simulink model "Fake_Algorithm_Control"  (Simulink 7.5)
settings: Solver=ode45  StartTime=0.0  StopTime=10.0  RelTol=1e-3
undefined symbols (not defined in the file): ctrller
settings Model: Creator=sriddle  LastModifiedBy=sriddle

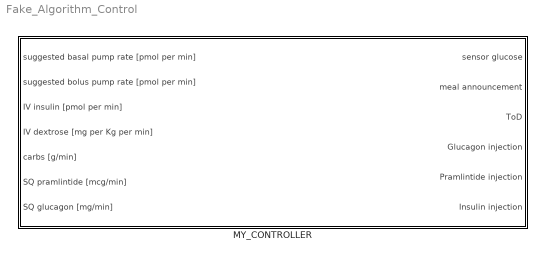
== system Fake_Algorithm_Control ==
  MY_CONTROLLER : Subsystem

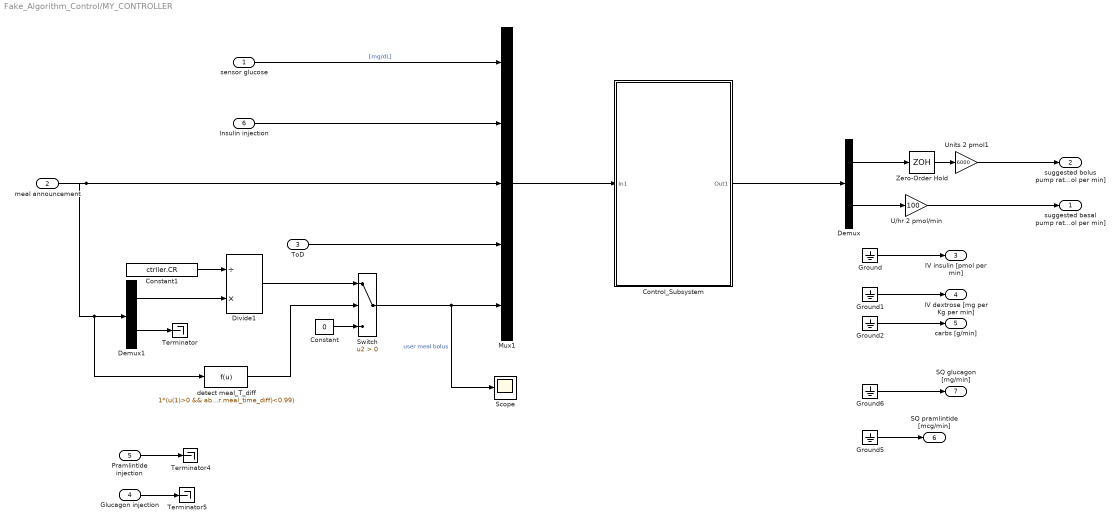
== system Fake_Algorithm_Control/MY_CONTROLLER ==
  sensor glucose : Inport  OutDataType=sfix(16)  OutScaling=2^0
  meal announcement : Inport  Port=2  OutDataType=sfix(16)  OutScaling=2^0
  ToD : Inport  Port=3  OutDataType=sfix(16)  OutScaling=2^0
  Glucagon injection : Inport  Port=4
  Pramlintide injection : Inport  Port=5
  Insulin injection : Inport  Port=6  OutDataType=sfix(16)  OutScaling=2^0
  Constant : Constant  Value=0  OutDataType=sfix(16)  OutScaling=2^0
  Constant1 : Constant  Value=ctrller.CR  OutDataType=sfix(16)  OutScaling=2^0
  Control_Subsystem : Subsystem
  Demux : Demux  Outputs=2
  Demux1 : Demux  Outputs=2
  Divide1 : Product  Inputs=/*  OutDataType=sfix(16)  OutScaling=2^-10
  Ground{,1..2,5..6} (5 alike) : Ground
  Mux1 : Mux  Inputs=5
  Scope : Scope
  Switch : Switch  Criteria=u2 > Threshold  OutDataType=sfix(16)  OutScaling=2^0
  Terminator : Terminator
  Terminator4 : Terminator
  Terminator5 : Terminator
  U/hr 2 pmol/min : Gain  Gain=100  ParameterDataType=sfix(16)  ParameterScaling=2^0  OutDataType=sfix(16)  OutScaling=2^0
  Units 2 pmol1 : Gain  Gain=6000  ParameterDataType=sfix(16)  ParameterScaling=2^0  OutDataType=sfix(16)  OutScaling=2^0
  Zero-Order Hold : ZeroOrderHold  SampleTime=-1
  detect meal_T_diff : Fcn  Expr=1*(u(1)>0 && abs(u(2)+ctrller.meal_time_diff)<0.99)
  suggested basal pump rate [pmol per min] : Outport  OutDataType=sfix(16)  OutScaling=2^0
  suggested bolus pump rate [pmol per min] : Outport  Port=2  OutDataType=sfix(16)  OutScaling=2^0
  IV insulin [pmol per min] : Outport  Port=3  OutDataType=sfix(16)  OutScaling=2^0
  IV dextrose [mg per Kg per min] : Outport  Port=4  OutDataType=sfix(16)  OutScaling=2^0
  carbs [g/min] : Outport  Port=5  OutDataType=sfix(16)  OutScaling=2^0
  SQ pramlintide [mcg/min] : Outport  Port=6
  SQ glucagon [mg/min] : Outport  Port=7
  wires:
  Demux/1 -> Zero-Order Hold/1
  Demux/2 -> U/hr 2 pmol/min/1
  ToD/1 -> Mux1/4
  sensor glucose/1 -> Mux1/1  "[mg/dL]"
  Insulin injection/1 -> Mux1/2
  Zero-Order Hold/1 -> Units 2 pmol1/1
  Constant1/1 -> Divide1/1
  Demux1/1 -> Divide1/2
  Constant/1 -> Switch/3
  Divide1/1 -> Switch/1
  Switch/1 -> Mux1/5, Scope/1  "user meal bolus"
  U/hr 2 pmol/min/1 -> suggested basal pump rate [pmol per min]/1
  meal announcement/1 -> Mux1/3, Demux1/1, detect meal_T_diff/1
  Ground2/1 -> carbs [g/min]/1
  Ground1/1 -> IV dextrose [mg per Kg per min]/1
  Ground/1 -> IV insulin [pmol per min]/1
  Units 2 pmol1/1 -> suggested bolus pump rate [pmol per min]/1
  Demux1/2 -> Terminator/1
  detect meal_T_diff/1 -> Switch/2
  Mux1/1 -> Control_Subsystem/1(In1)
  Control_Subsystem/1(Out1) -> Demux/1
  Pramlintide injection/1 -> Terminator4/1
  Glucagon injection/1 -> Terminator5/1
  Ground6/1 -> SQ glucagon [mg/min]/1
  Ground5/1 -> SQ pramlintide [mcg/min]/1

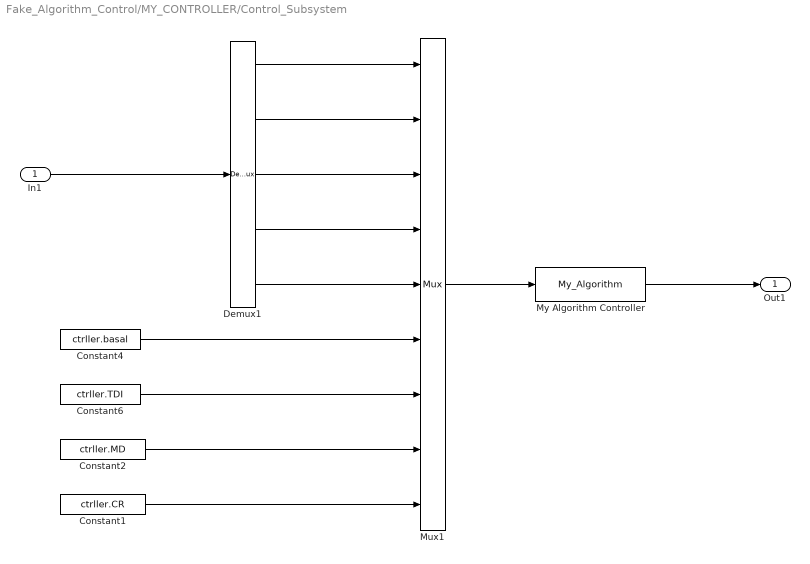
== system Fake_Algorithm_Control/MY_CONTROLLER/Control_Subsystem ==
  In1 : Inport  OutDataType=fixdt(1, 16)  OutScaling=2^0
  Constant1 : Constant  Value=ctrller.CR
  Constant2 : Constant  Value=ctrller.MD
  Constant4 : Constant  Value=ctrller.basal
  Constant6 : Constant  Value=ctrller.TDI
  Demux1 : Demux  Outputs=5
  Mux1 : Mux  Inputs=9
  My Algorithm Controller : S-Function  FunctionName=My_Algorithm  EnableBusSupport=off
  Out1 : Outport  OutDataType=fixdt(1, 16)  OutScaling=2^0
  wires:
  Demux1/5 -> Mux1/5
  Demux1/4 -> Mux1/4
  Demux1/3 -> Mux1/3
  Demux1/2 -> Mux1/2
  Demux1/1 -> Mux1/1
  In1/1 -> Demux1/1
  Constant1/1 -> Mux1/9
  Constant2/1 -> Mux1/8
  Constant6/1 -> Mux1/7
  Constant4/1 -> Mux1/6
  Mux1/1 -> My Algorithm Controller/1
  My Algorithm Controller/1 -> Out1/1
